simulink library "saturate_rwa_lib"  (R2018b)
settings: Solver=VariableStepAuto  StartTime=0.0  StopTime=10.0  RelTol=1e-3
undefined symbols (not defined in the file or in its folder): fswParams
libraries: simulink x1
settings Model: Creator=taylorreynolds  LastModifiedBy=taylorreynolds

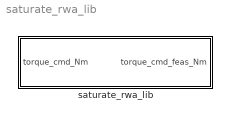
== system saturate_rwa_lib ==
  saturate_rwa_lib : Subsystem  TreatAsAtomicUnit=on
      settings: RTWFcnNameOpts=Use subsystem name  RTWFileNameOpts=Use subsystem name

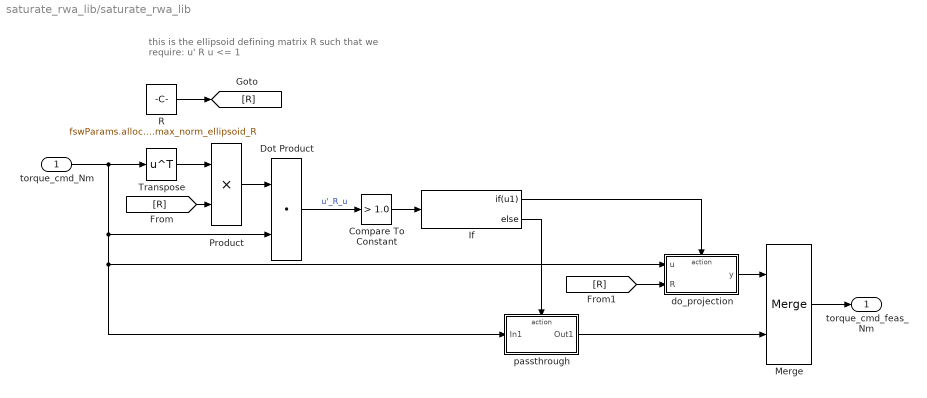
== system saturate_rwa_lib/saturate_rwa_lib ==
  note: this is the ellipsoid defining matrix R
      | such that we require:
      | u' R u <= 1
  torque_cmd_Nm : Inport
  Compare To Constant : simulink/Logic and Bit Operations/Compare To Constant  relop=>  const=1.0  OutDataTypeStr=boolean
  Dot Product : DotProduct  InputSameDT=on  OutDataTypeStr=Inherit: Inherit via internal rule
  If : If  IfExpression=u1
  Merge : Merge
  Product : Product
  R : Constant  Value=fswParams.allocator.rwa.max_norm_ellipsoid_R
  Transpose : Math  Operator=transpose  SaturateOnIntegerOverflow=on
  do_projection : Subsystem  TreatAsAtomicUnit=on
  passthrough : Subsystem  TreatAsAtomicUnit=on
  torque_cmd_feas_Nm : Outport
  wires:
  torque_cmd_Nm/1 -> passthrough/1(In1), do_projection/1(u), Dot Product/2, Transpose/1
  Transpose/1 -> Product/1
  Product/1 -> Dot Product/1
  Dot Product/1 -> Compare To Constant/1  "u'_R_u"
  Compare To Constant/1 -> If/1
  If/1 -> do_projection/Action
  If/2 -> passthrough/Action
  do_projection/1(y) -> Merge/1
  passthrough/1(Out1) -> Merge/2
  Merge/1 -> torque_cmd_feas_Nm/1
  R/1 -> [R]
  [R] -> Product/2
  [R] -> do_projection/2(R)

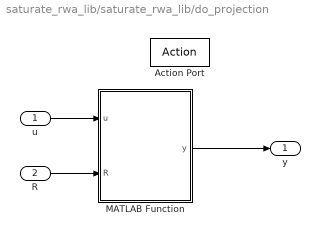
== system saturate_rwa_lib/saturate_rwa_lib/do_projection ==
  u : Inport
  R : Inport  Port=2
  Action Port : ActionPort  ActionType=then
  MATLAB Function : MATLAB Function  TreatAsAtomicUnit=on
  y : Outport
  wires:
  u/1 -> MATLAB Function/1(u)
  R/1 -> MATLAB Function/2(R)
  MATLAB Function/1(y) -> y/1

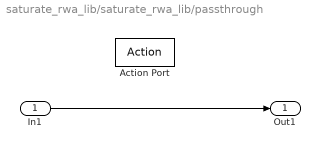
== system saturate_rwa_lib/saturate_rwa_lib/passthrough ==
  In1 : Inport
  Action Port : ActionPort  ActionType=else
  Out1 : Outport
  wires:
  In1/1 -> Out1/1

== matlab function saturate_rwa_lib/do_projection/MATLAB Function ==
  data: u input size=3; y output size=3; R input size=3
function y = project_onto_ellip(u,R)
%PROJECT_ONTO_ELLIP
%
% Returns the projection of u onto the ellipsoid R, defined as the solution
% to the optimization problem
%
%   y = argmin_x ||x-u||^2
%   s.t. x'*R*x <= 1
%
% The solution is given by
%   x = ( lambda*R + I ) \ u
% for the (strictly positive) Lagrange multiplier lambda. This function
% uses Newton's method to iteratively find the value of lambda so that x
% lies on the boundary of the ellipsoid, ie. x'*R*x == 1. 
%
% Assumes that R is a diagonal matrix stored as a 3x1 column vector. Most
% of the mathematics have been boiled down using this fact, so matrix
% products like x=(lambda*R+I)\u are written like
%   x_i = u_i/(lambda*R_i+1.0),  i = 1,2,3
%
% T. Reynolds -- May 11, 2020
%#codegen

% constants
tol = 1e-5;
max_iter = uint32(10);

% compute initial guess
lambda = 0.0;
x = [ u(1)/(lambda*R(1)+1.0);
      u(2)/(lambda*R(2)+1.0);
      u(3)/(lambda*R(3)+1.0) ];

% main loop
for iter = 1:max_iter
    
    % current function value
    g = x'*(R.*x) - 1;
    if (abs(g)<tol)
        y = x;
        return;
    end
    
    % current derivative value
    A = [ R(1)/(lambda*R(1)+1.0);
          R(2)/(lambda*R(2)+1.0);
          R(3)/(lambda*R(3)+1.0) ].^2;
    dg = -2.0 * dot(x, A.*u);
    
    % update multiplier
    lambda_new = lambda - g/dg;
    
    % update solution
    x_new = [ u(1)/(lambda_new*R(1)+1.0);
              u(2)/(lambda_new*R(2)+1.0);
              u(3)/(lambda_new*R(3)+1.0) ];
    
    % check convergence
    if (norm(x-x_new)<tol)
        y = x_new;
        return;
    end
    
    % update parameters
    lambda = lambda_new;
    x = x_new;  
end
% if we did not converge in the allotted number of iterations, output the
% current guess
y = x;
end
